simulink model "model_SEIRD_LlitsUCI"  (R2023a)
settings: Solver=VariableStepAuto  StartTime=0.0  StopTime=365  RelTol=1e-3
model workspace (MAT data in the model file):
  b = 0.3
  d = 0.02
  g = 0.1
  l = 0.2
  n = 7500000
  ratio_hosp = 0.05
settings Model: Creator=joans  LastModifiedBy=joans
settings SolverCC: ZeroCrossControl=DisableAll
settings ModelReferenceCC: EnableRefExpFcnMdlSchedulingChecks=on

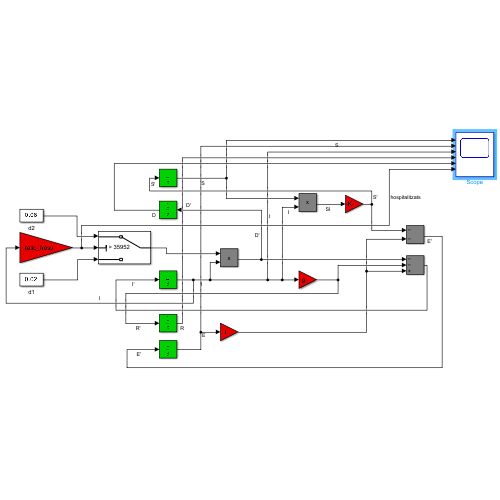
[thumbnail: Simulink's stored preview of the top-level diagram]
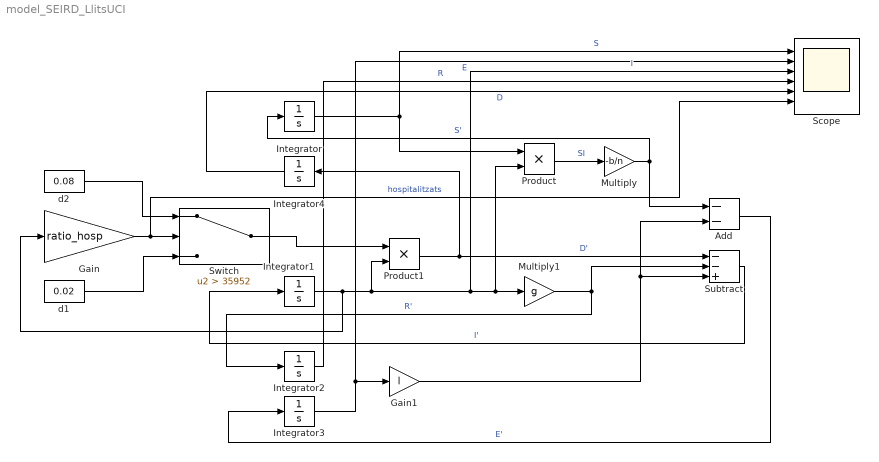
== system model_SEIRD_LlitsUCI ==
  Add : Sum  Inputs=--
  Gain : Gain  Gain=ratio_hosp
  Gain1 : Gain  Gain=l
  Integrator : Integrator  InitialCondition=n
  Integrator1 : Integrator  InitialCondition=10
  Integrator2 : Integrator
  Integrator3 : Integrator
  Integrator4 : Integrator
  Multiply : Gain  Gain=-b/n
  Multiply1 : Gain  Gain=g
  Product : Product
  Product1 : Product
  Scope : Scope  NumInputPorts=6
  Subtract : Sum  Inputs=--+
  Switch : Switch  Criteria=u2 > Threshold  Threshold=35952  SaturateOnIntegerOverflow=off  InputSameDT=off
  d1 : Constant  Value=0.02
  d2 : Constant  Value=0.08
  wires:
  Integrator/1 -> Product/1, Scope/1  "S"
  Integrator1/1 -> Gain/1, Product/2, Multiply1/1, Scope/3, Product1/2  "I"
  Product/1 -> Multiply/1  "SI"
  Multiply/1 -> Add/1, Integrator/1  "S'"
  Multiply1/1 -> Integrator2/1, Subtract/2  "R'"
  Integrator2/1 -> Scope/4  "R"
  Integrator3/1 -> Scope/2, Gain1/1  "E"
  Subtract/1 -> Integrator1/1  "I'"
  Integrator4/1 -> Scope/5  "D"
  Product1/1 -> Integrator4/1, Subtract/1  "D'"
  Gain1/1 -> Subtract/3, Add/2
  Add/1 -> Integrator3/1  "E'"
  Switch/1 -> Product1/1
  d2/1 -> Switch/1
  d1/1 -> Switch/3
  Gain/1 -> Switch/2, Scope/6  "hospitalitzats"
